simulink model "Lowpass"  (R2021b)
settings: Solver=VariableStepAuto  StartTime=0.0  StopTime=10.0  RelTol=1e-3
undefined symbols (not defined in the file): fdesignblkfcn, gcbh
libraries: dspsigops x2, dspsnks4 x1, dspvision x1
settings Model: Creator=leemuhera  LastModifiedBy=leemuhera

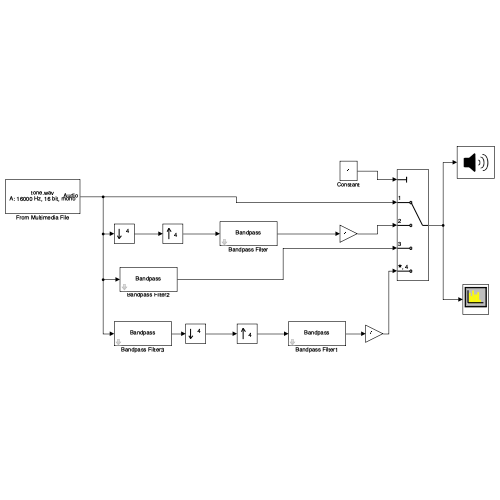
[thumbnail: Simulink's stored preview of the top-level diagram]
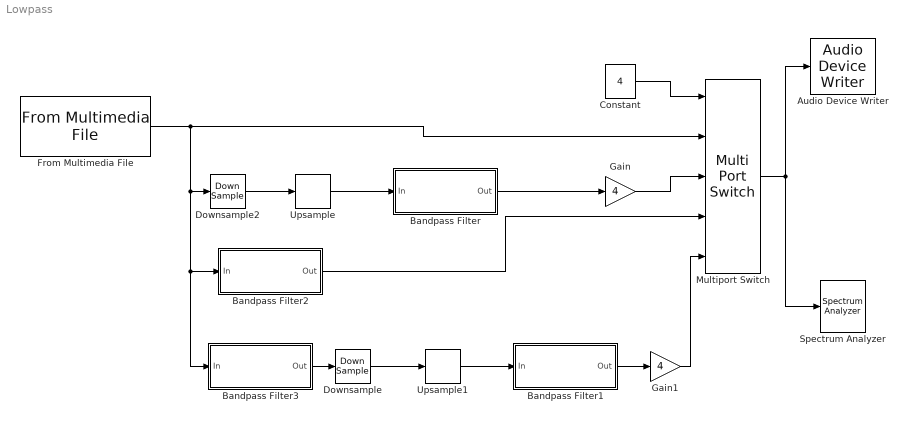
== system Lowpass ==
  Audio Device Writer : dspsnks4/Audio Device Writer  Driver=CoreAudio  Device=Built-in Output  InheritSampleRate=on  SampleRate=44100  BitDepth=16-bit integer  BufferSize=4096  NumBuffers=10  DefaultOutputChannelMapping=on  OutputChannelMapping=1:2  OutputNumUnderrunSamples=off  DriverIdx=5  DeviceWarnFlag=''
  Bandpass Filter : Subsystem  DialogController=fdesignblkfcn  InitFcn=fdesignblkfcn(gcbh, {'InitFcn'});  mask(Bandpass Filter){}
      mask help: Design a bandpass filter
      settings: CopyFcn=fdesignblkfcn(gcbh, {'CopyFcn'});
      mask Help: helpview(mapfilelocation('dsp'), 'dspbandpassfilter');
      mask Display: disp('Bandpass');
  Bandpass Filter1 : Subsystem  DialogController=fdesignblkfcn  InitFcn=fdesignblkfcn(gcbh, {'InitFcn'});  mask(Bandpass Filter){}
      mask help: Design a bandpass filter
      settings: CopyFcn=fdesignblkfcn(gcbh, {'CopyFcn'});
      mask Help: helpview(mapfilelocation('dsp'), 'dspbandpassfilter');
      mask Display: disp('Bandpass');
  Bandpass Filter2 : Subsystem  DialogController=fdesignblkfcn  InitFcn=fdesignblkfcn(gcbh, {'InitFcn'});  mask(Bandpass Filter){}
      mask help: Design a bandpass filter
      settings: CopyFcn=fdesignblkfcn(gcbh, {'CopyFcn'});
      mask Help: helpview(mapfilelocation('dsp'), 'dspbandpassfilter');
      mask Display: disp('Bandpass');
  Bandpass Filter3 : Subsystem  DialogController=fdesignblkfcn  InitFcn=fdesignblkfcn(gcbh, {'InitFcn'});  mask(Bandpass Filter){}
      mask help: Design a bandpass filter
      settings: CopyFcn=fdesignblkfcn(gcbh, {'CopyFcn'});
      mask Help: helpview(mapfilelocation('dsp'), 'dspbandpassfilter');
      mask Display: disp('Bandpass');
  Constant : Constant  Value=4  VectorParams1D=off
  Downsample : DownSample  N=4
  Downsample2 : DownSample  N=4
  From Multimedia File : dspvision/From Multimedia File  inputFilename=/Users/leemuhera/Documents/DSP Lab /Lab 3/tone.wav  readRange=[1 Inf]  loop=on  numPlays=inf  outputStreams=Audio only  videoDataType=single  audioDataType=double  inheritSampleTime=on  userDefinedSampleTime=1/30  noAudioOutput=off  isIntensityVideo=off  fourcc=RGB  colorVideoFormat=Separate color signals  outputEOF=off  dataOrg=Column-major  audioFrameSize=1024  computeAudioFrameSize=off  outSamplingMode=Sample based
  Gain : Gain  Gain=4
  Gain1 : Gain  Gain=4
  Multiport Switch : MultiPortSwitch  Inputs=4
  Spectrum Analyzer : SpectrumAnalyzer
  Upsample : dspsigops/Upsample  N=4  phase=0  InputProcessing=Columns as channels (frame based)  RateOptions=Enforce single-rate processing  ic=0  mode=Unused parameter value
  Upsample1 : dspsigops/Upsample  N=4  phase=0  InputProcessing=Columns as channels (frame based)  RateOptions=Enforce single-rate processing  ic=0  mode=Unused parameter value
  wires:
  From Multimedia File/1 -> Downsample2/1, Bandpass Filter3/1(In), Bandpass Filter2/1(In), Multiport Switch/2
  Downsample2/1 -> Upsample/1
  Bandpass Filter/1(Out) -> Gain/1
  Gain/1 -> Multiport Switch/3
  Constant/1 -> Multiport Switch/1
  Bandpass Filter2/1(Out) -> Multiport Switch/4
  Downsample/1 -> Upsample1/1
  Upsample1/1 -> Bandpass Filter1/1(In)
  Gain1/1 -> Multiport Switch/5
  Multiport Switch/1 -> Audio Device Writer/1, Spectrum Analyzer/1
  Bandpass Filter1/1(Out) -> Gain1/1
  Bandpass Filter3/1(Out) -> Downsample/1
  Upsample/1 -> Bandpass Filter/1(In)

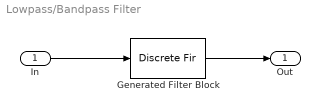
== system Lowpass/Bandpass Filter ==
  In : Inport
  Generated Filter Block : DiscreteFir  Tag=BlockMethodSubSystem  Coefficients=[-0.0008992291487744296 0.0016414518747943749 0.0031352071842225397 -0.0040707550828814922 -0.0063731852227904111 0.0074874286806090491 0.0098354319566295711 -0.010189316513446216 -0.011302794465874122 0.0096929185841818435 0.0079428653987464216 -0.0031368247881221642 0.0028299878877943137 -0.011508674243001471 -0.022080136219461581 0.034245325424507672 0.048356661648905473 -0.062355369169884239 -0.077503478162593897 0.090687768153125653 0.10353171105844157 -0.11297860084229834 -0.12035866024978455 0.12379360801539134 0.12379360801539134 -0.12035866024978455 -0.11297860084229834 0.10353171105844157 0.090687768153125653 -0.077503478162593897 -0.062355369169884239 0.048356661648905473 0.034245325424507672 -0.022080136219461581 -0.011508674243001471 0.0028299878877943137 -0.0031368247881221642 0.0079428653987464216 0.0096929185841818435 -0.011302794465874122 -0.010189316513446216 0.0098354319566295711 0.0074874286806090491 -0.0063731852227904111 -0.0040707550828814922 0.0031352071842225397 0.0016414518747943749 -0.0008992291487744296]  InputProcessing=Columns as channels (frame based)
  Out : Outport  VectorParamsAs1DForOutWhenUnconnected=off
  wires:
  In/1 -> Generated Filter Block/1
  Generated Filter Block/1 -> Out/1

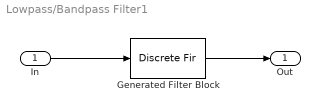
== system Lowpass/Bandpass Filter1 ==
  In : Inport
  Generated Filter Block : DiscreteFir  Tag=BlockMethodSubSystem  Coefficients=[-0.0008992291487744296 0.0016414518747943749 0.0031352071842225397 -0.0040707550828814922 -0.0063731852227904111 0.0074874286806090491 0.0098354319566295711 -0.010189316513446216 -0.011302794465874122 0.0096929185841818435 0.0079428653987464216 -0.0031368247881221642 0.0028299878877943137 -0.011508674243001471 -0.022080136219461581 0.034245325424507672 0.048356661648905473 -0.062355369169884239 -0.077503478162593897 0.090687768153125653 0.10353171105844157 -0.11297860084229834 -0.12035866024978455 0.12379360801539134 0.12379360801539134 -0.12035866024978455 -0.11297860084229834 0.10353171105844157 0.090687768153125653 -0.077503478162593897 -0.062355369169884239 0.048356661648905473 0.034245325424507672 -0.022080136219461581 -0.011508674243001471 0.0028299878877943137 -0.0031368247881221642 0.0079428653987464216 0.0096929185841818435 -0.011302794465874122 -0.010189316513446216 0.0098354319566295711 0.0074874286806090491 -0.0063731852227904111 -0.0040707550828814922 0.0031352071842225397 0.0016414518747943749 -0.0008992291487744296]  InputProcessing=Columns as channels (frame based)
  Out : Outport  VectorParamsAs1DForOutWhenUnconnected=off
  wires:
  In/1 -> Generated Filter Block/1
  Generated Filter Block/1 -> Out/1

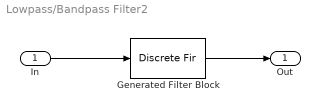
== system Lowpass/Bandpass Filter2 ==
  In : Inport
  Generated Filter Block : DiscreteFir  Tag=BlockMethodSubSystem  Coefficients=[-0.0008992291487744296 0.0016414518747943749 0.0031352071842225397 -0.0040707550828814922 -0.0063731852227904111 0.0074874286806090491 0.0098354319566295711 -0.010189316513446216 -0.011302794465874122 0.0096929185841818435 0.0079428653987464216 -0.0031368247881221642 0.0028299878877943137 -0.011508674243001471 -0.022080136219461581 0.034245325424507672 0.048356661648905473 -0.062355369169884239 -0.077503478162593897 0.090687768153125653 0.10353171105844157 -0.11297860084229834 -0.12035866024978455 0.12379360801539134 0.12379360801539134 -0.12035866024978455 -0.11297860084229834 0.10353171105844157 0.090687768153125653 -0.077503478162593897 -0.062355369169884239 0.048356661648905473 0.034245325424507672 -0.022080136219461581 -0.011508674243001471 0.0028299878877943137 -0.0031368247881221642 0.0079428653987464216 0.0096929185841818435 -0.011302794465874122 -0.010189316513446216 0.0098354319566295711 0.0074874286806090491 -0.0063731852227904111 -0.0040707550828814922 0.0031352071842225397 0.0016414518747943749 -0.0008992291487744296]  InputProcessing=Columns as channels (frame based)
  Out : Outport  VectorParamsAs1DForOutWhenUnconnected=off
  wires:
  In/1 -> Generated Filter Block/1
  Generated Filter Block/1 -> Out/1

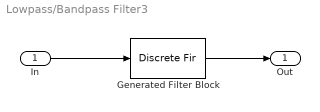
== system Lowpass/Bandpass Filter3 ==
  In : Inport
  Generated Filter Block : DiscreteFir  Tag=BlockMethodSubSystem  Coefficients=[-0.0008992291487744296 0.0016414518747943749 0.0031352071842225397 -0.0040707550828814922 -0.0063731852227904111 0.0074874286806090491 0.0098354319566295711 -0.010189316513446216 -0.011302794465874122 0.0096929185841818435 0.0079428653987464216 -0.0031368247881221642 0.0028299878877943137 -0.011508674243001471 -0.022080136219461581 0.034245325424507672 0.048356661648905473 -0.062355369169884239 -0.077503478162593897 0.090687768153125653 0.10353171105844157 -0.11297860084229834 -0.12035866024978455 0.12379360801539134 0.12379360801539134 -0.12035866024978455 -0.11297860084229834 0.10353171105844157 0.090687768153125653 -0.077503478162593897 -0.062355369169884239 0.048356661648905473 0.034245325424507672 -0.022080136219461581 -0.011508674243001471 0.0028299878877943137 -0.0031368247881221642 0.0079428653987464216 0.0096929185841818435 -0.011302794465874122 -0.010189316513446216 0.0098354319566295711 0.0074874286806090491 -0.0063731852227904111 -0.0040707550828814922 0.0031352071842225397 0.0016414518747943749 -0.0008992291487744296]  InputProcessing=Columns as channels (frame based)
  Out : Outport  VectorParamsAs1DForOutWhenUnconnected=off
  wires:
  In/1 -> Generated Filter Block/1
  Generated Filter Block/1 -> Out/1
